simulink model "W07_C_wave"  (R2024b)
settings: Solver=ode4  StartTime=0  StopTime=T_final  FixedStep=h  RelTol=1e-3
values from neighbouring files (symbols this model uses):
  wave_on = 1    [W07_0_setup.m]
undefined symbols (not defined in the file or in its folder): a_i, k_w, phi_i, w_i
settings Model: Creator=admin  LastModifiedBy=admin
settings DataIOCC: ReturnWorkspaceOutputs=off

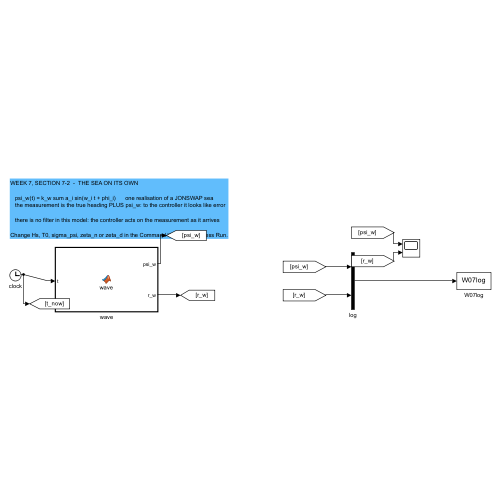
[thumbnail: Simulink's stored preview of the top-level diagram]
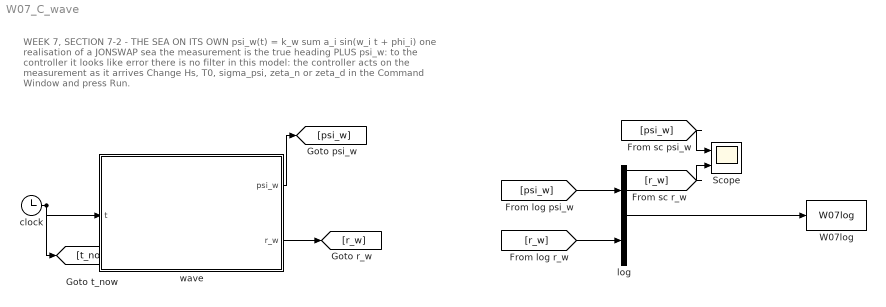
== system W07_C_wave ==
  note: WEEK 7, SECTION 7-2  -  THE SEA ON ITS OWN
      |
      |    psi_w(t) = k_w sum a_i sin(w_i t + phi_i)      one realisation of a JONSWAP sea
      |    the measurement is the true heading PLUS psi_w: to the controller it looks like error
      |
      |    there is no filter in this model: the controller acts on the measurement as it arrives
      |
      | Change Hs, T0, sigma_psi, zeta_n or zeta_d in the Command Window and press Run.
  Scope : Scope  NumInputPorts=2
  W07log : ToWorkspace  VariableName=W07log  SaveFormat=Structure With Time  SampleTime=-1
  clock : Clock
  log : Mux  Inputs=2
  wave : MATLAB Function  TreatAsAtomicUnit=on
  wires:
  clock/1 -> wave/1(t), [t_now]
  wave/1(psi_w) -> [psi_w]
  wave/2(r_w) -> [r_w]
  [psi_w] -> log/1
  [psi_w] -> Scope/1
  [r_w] -> log/2
  [r_w] -> Scope/2
  log/1 -> W07log/1

== matlab function W07_C_wave/wave ==
  data: t input; psi_w output double size=[1 1]; r_w output; w_i parameter; a_i parameter; phi_i parameter; k_w parameter; wave_on parameter
function [psi_w, r_w] = wave(t, w_i, a_i, phi_i, k_w, wave_on)
%#codegen
%  1차 파랑이 만드는 선수각과 그 변화율 / the wave-induced heading and its rate
%
%  스펙트럼 하나를 성분 여럿의 합으로 적는다. 진폭은 JONSWAP 에서 나오고 (wave_train),
%  위상은 정해져 있으므로 이 바다는 매번 똑같다 — 강의의 표를 재현할 수 있다.
%  One spectrum, written as a sum of components: the amplitudes come from JONSWAP
%  and the phases are fixed, so this sea is the same on every run.
%
%      psi_w(t) = k_w * sum_i a_i sin(w_i t + phi_i)          [deg]
%      r_w(t)   = k_w * sum_i a_i w_i cos(w_i t + phi_i)      [deg/s]
%
%  k_w 는 진폭 [m] 을 선수각 [deg] 으로 바꾸는 배율이다. 이 주차는 그 응답을
%  유도하지 않고 **주어진 것으로** 둔다 — 표준편차 sigma_psi 로 적는다.
%  k_w turns a wave amplitude into a heading. This week does not derive that
%  response; it takes it as given, stated by its standard deviation.
psi_w = 0;  r_w = 0;
if wave_on ~= 0
    for i = 1:numel(w_i)
        psi_w = psi_w + k_w*a_i(i)*sin(w_i(i)*t + phi_i(i));
        r_w   = r_w   + k_w*a_i(i)*w_i(i)*cos(w_i(i)*t + phi_i(i));
    end
end
